simulink model "sm_worm_jack"  (R2021b)
settings: Solver=ode15s  StartTime=0.0  StopTime=15  MaxStep=0.01  RelTol=1e-3  EnableMultiTasking=on
model workspace: external: MATLAB File sm_worm_jack_parameters.m (data not in the file)
values from neighbouring files (symbols this model uses):
  ctrlStepTime = 5    [sm_worm_jack_parameters.m]
undefined symbols (not defined in the file or in its folder): jack, X, Y, Z
libraries: nesl_utility x5, sm_worm_jack_lib x4, sm_lib x3
settings Model: Creator=The MathWorks, Inc.  LastModifiedBy=The MathWorks, Inc.
settings SolverCC: AlgebraicLoopSolver=TrustRegion
settings DataIOCC: LimitDataPoints=on  ReturnWorkspaceOutputs=off
settings OptimizationCC: LifeSpan=inf
settings DebuggingCC: AllowSymbolicDim=off  SFUnexpectedBacktrackingDiag=warning  SFNoUnconditionalDefaultTransitionDiag=warning  SFExecutionAtInitializationDiag=none  SFMachineParentedDataDiag=warning  ArithmeticOperatorsInVariantConditions=warning
settings SFSimCC: SimUseLocalCustomCode=off  CustomCodeUndefinedFunction=UseInterfaceOnly
settings RTWCC: RTWUseLocalCustomCode=off
settings CodeAppCC: StateflowObjectComments=on
settings GRTTargetCC: TargetLangStandard=C89/C90 (ANSI)
settings ConfigComp: CovMetricSettings=dw  CovSaveCumulativeToWorkspaceVar=on  CovSaveSingleToWorkspaceVar=on  CovExternalEMLEnable=off  CovSFcnEnable=off
settings SimscapeCC: SimscapeNormalizeSystem=off  SimscapeLogType=all  SimscapeLogSimulationStatistics=on  SimscapeLogName=simlog_sm_worm_jack  SimscapeLogDataHistory=10000
settings ConfigurationSet: Description=SimMechanics 2G
settings ExplorerConfigSet: InternalSimMechanicsExplorerSettings="<ExplorerConfiguration><canonicalview>default</canonicalview><AnimationSetting><BasePlaybackSpeed>1.0</BasePlaybackSpeed><PlaybackSpeedFactor>1.0</PlaybackSpeedFactor></AnimationSetting><TilePanel><TileInfo><Tiles Columns=\"1\" Count=\"1\" Rows=\"1\"><Column Weight=\"1\"/><Row Weight=\"1\"/><Tile Height=\"1\" Width=\"1\" X=\"0\" Y=\"0\"/></Tiles></TileInfo><SceneInfo><SceneViewer><BGColor><R>0.60000002384185791</R><G>0.60000002384185791</G><B>0.60000002384185791</B></BGColor><Camera><DoPerspective>off</DoPerspective><Position><X>0.643732116535259746</X><Y>-0.308018560744014402</Y><Z>0.64842413062973181</Z></Position><Center><X>0.0663818473456340569</X><Y>0.269331708445611495</Y><Z>0.0710738614401060786</Z></Center><Up><X>-0.408248290463863073</X><Y>0.408248290463863073</Y><Z>0.816496580927726145</Z></Up><ViewLimDist>1</ViewLimDist><YLim>0.376296170188444967</YLim><XLim>0.50655253679213752</XLim></Camera></SceneViewer></SceneInfo></TilePanel><MechEditorPanel><Cameras/><GfxPanelCameraMap/><VideoCreator><PlaybackSpeedRatio>1.0</PlaybackSpeedRatio><FrameRate>30</FrameRate><VideoFormat>Motion JPEG AVI</VideoFormat><FrameSize>auto</FrameSize></VideoCreator></MechEditorPanel></ExplorerConfiguration>"

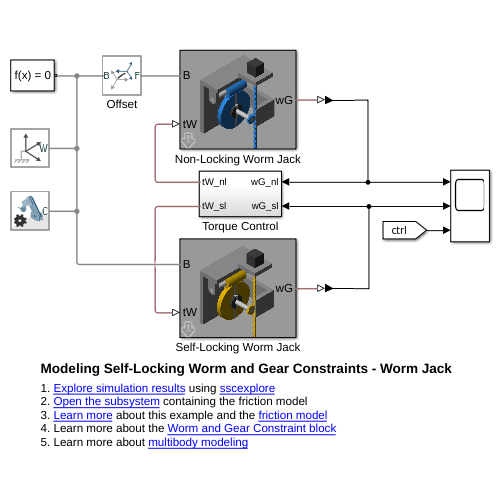
[thumbnail: Simulink's stored preview of the top-level diagram]
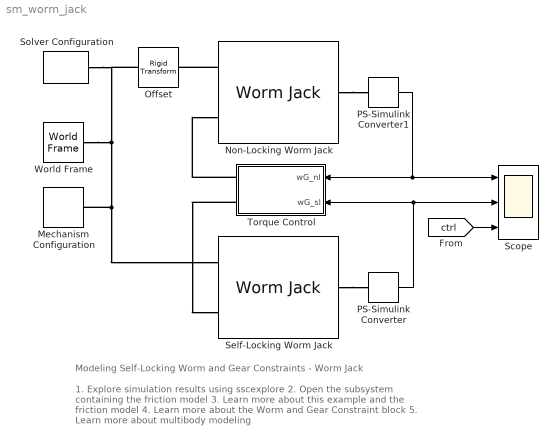
== system sm_worm_jack ==
  note: 1. Explore simulation results using sscexplore
      | 2. Open the subsystem containing the friction model
      | 3. Learn more about this example and the friction model
      | 4. Learn more about the Worm and Gear Constraint block
      | 5. Learn more about multibody modeling
  note: Modeling Self-Locking Worm and Gear Constraints - Worm Jack
  Mechanism Configuration : sm_lib/Utilities/Mechanism Configuration  UniformGravity=Constant  GravityVector=[0 0 -9.80665]  GravityUnits=m/s^2  LinearizationDelta=0.001  JointModeTransitionNonlinearIterations=2
  Non-Locking Worm Jack : sm_worm_jack_lib/Worm Jack  wormLeadAngle=nonlock.wormLeadAngle  wormRadius=jack.wormRadius  wormLength=jack.wormLength  wormShaftLength=jack.wormShaftLength  gearRadius=jack.gearRadius  gearLength=jack.gearLength  gearShaftLength=jack.gearShaftLength  collarRadius=jack.collarRadius  shaftRadius=jack.shaftRadii  rackLength=jack.rackLength  pinionRadius=jack.pinionRadius  pinionTeeth=jack.pinionTeeth  pinionShaftLength=jack.pinionShaft  loadWidth=jack.loadWidth  plateThickness=jack.plateThickness  wG_0=jack.gearRevolute_w0  muK=jack.kineticFriction  muS=jack.staticFriction  vth=jack.velocityThreshold  t_c=jack.filterConstant  wormRho=jack.wormDensity  gearRho=jack.gearDensity  shaftRho=jack.shaftDensity  collarRho=jack.collarDensity  rackRho=jack.rackDensity  pinionRho=jack.pinionDensity  housingRho=jack.housingDensity  boxRho=jack.boxDensity  wormColor=nonlock.wormColor  gearColor=nonlock.gearColor  shaftColor=jack.shaftColor  collarColor=jack.collarColor  rackColor=nonlock.rackColor  pinionColor=nonlock.pinionColor  housingColor=jack.housingColor  boxColor=jack.boxColor  sliceColor=jack.sliceColor  mask(Worm Drive Assembly){}
      settings: SourceProductBaseCode=MS
      mask Display:
      | image(imread(fullfile(matlabroot,'toolbox','physmod','sm','smdemos','worm_jack','images','sm_worm_jack_nonlocking_wormjack.png')));
      | port_label('lconn',1,'B');
      | port_label('lconn',2,'tW');
      | port_label('rconn',1,'wG');
  Offset : sm_lib/Frames and Transforms/Rigid Transform  TranslationMethod=StandardAxis  TranslationStandardOffset=nonlock.offset  TranslationLengthUnit=m  TranslationStandardAxis=+Y  TranslationCartesianOffset=0  TranslationROffset=0  TranslationROffsetUnits=m  TranslationZOffset=0  TranslationZOffsetUnits=m  TranslationThetaOffset=0  TranslationThetaOffsetUnits=deg  RotationMethod=None  RotationAngleUnits=deg  RotationStandardAxis=+Z  RotationAngle=0.0  RotationArbitraryAxis=[0 0 1]  FollAlignAxisA=+X  BaseAlignAxisA=+Y  FollAlignAxisB=+Y  BaseAlignAxisB=+Z  RotationSequenceAxes=FollowerAxes  RotationSequence=XYX  RotationSequenceAngles=[0 0 0]  RotationSequenceAnglesUnits=deg  RotationMatrix=[1 0 0; 0 1 0; 0 0 1]
  PS-Simulink Converter : nesl_utility/PS-Simulink Converter  PhysicalDomain=network_engine_domain  SubClassName=ps_output  LeftPortType=input  RightPortType=output  PseudoPeriodic=off  Frequencies=[]  Unit=deg/s  AffineConversion=off
      settings: SourceProductBaseCode=PW,SS
  PS-Simulink Converter1 : nesl_utility/PS-Simulink Converter  PhysicalDomain=network_engine_domain  SubClassName=ps_output  LeftPortType=input  RightPortType=output  PseudoPeriodic=off  Frequencies=[]  Unit=deg/s  AffineConversion=off
      settings: SourceProductBaseCode=PW,SS
  Scope : Scope  NumInputPorts=3
  Self-Locking Worm Jack : sm_worm_jack_lib/Worm Jack  wormLeadAngle=selflock.wormLeadAngle  wormRadius=jack.wormRadius  wormLength=jack.wormLength  wormShaftLength=jack.wormShaftLength  gearRadius=jack.gearRadius  gearLength=jack.gearLength  gearShaftLength=jack.gearShaftLength  collarRadius=jack.collarRadius  shaftRadius=jack.shaftRadii  rackLength=jack.rackLength  pinionRadius=jack.pinionRadius  pinionTeeth=jack.pinionTeeth  pinionShaftLength=jack.pinionShaft  loadWidth=jack.loadWidth  plateThickness=jack.plateThickness  wG_0=jack.gearRevolute_w0  muK=jack.kineticFriction  muS=jack.staticFriction  vth=jack.velocityThreshold  t_c=jack.filterConstant  wormRho=jack.wormDensity  gearRho=jack.gearDensity  shaftRho=jack.shaftDensity  collarRho=jack.collarDensity  rackRho=jack.rackDensity  pinionRho=jack.pinionDensity  housingRho=jack.housingDensity  boxRho=jack.boxDensity  wormColor=selflock.wormColor  gearColor=selflock.gearColor  shaftColor=jack.shaftColor  collarColor=jack.collarColor  rackColor=selflock.rackColor  pinionColor=selflock.pinionColor  housingColor=jack.housingColor  boxColor=jack.boxColor  sliceColor=jack.sliceColor  mask(Worm Drive Assembly){}
      settings: SourceProductBaseCode=MS
      mask Display:
      | image(imread(fullfile(matlabroot,'toolbox','physmod','sm','smdemos','worm_jack','images','sm_worm_jack_selflocking_wormjack.png')));
      | port_label('lconn',1,'B');
      | port_label('lconn',2,'tW');
      | port_label('rconn',1,'wG');
  Solver Configuration : nesl_utility/Solver Configuration  PhysicalDomain=network_engine_domain  SubClassName=solver  LeftPortType=input  RightPortType=generic  Tones=[]  Harmonics=[]  SimulateNoise=off  Profile=off  UseLocalSampling=off  EnableSwitchedLinearOptims=on  FrequencyDomain=off  UseCCode=off  RelTol=0.001  AbsTol=1e-06  MinStep=1e-09  ToWorkspace=off  RevertToSquareIcSolve=off  NumHomotopyIterations=100  PhasorMode=off  PhasorModeNumHarmonics=1  DoDC=off  ResidualTolerance=1e-9  UseLocalSolver=off  LocalSolverChoice=NE_BACKWARD_EULER_ADVANCER  LocalSolverSampleTime=0.001  DoFixedCost=off  MaxNonlinIter=3  MaxModeIter=2  ComputeImpulses=off  ImpulseIterations=2  LinearAlgebra=Sparse  EquationFormulation=NE_TIME_EF  DelaysMemoryBudget=1024  AutomaticFiltering=on  FilteringTimeConstant=0.001  PartitionStorageMethod=AS_NEEDED  PartitionMemoryBudget=1024  PartitionMethod=FAST
      settings: SourceProductBaseCode=PW,SS
  Torque Control : Subsystem
  World Frame : sm_lib/Frames and Transforms/World Frame
  wires:
  PS-Simulink Converter1/1 -> Scope/1, Torque Control/1(wG_nl)
  PS-Simulink Converter/1 -> Scope/2, Torque Control/2(wG_sl)
  [ctrl] -> Scope/3
  connections:
  Non-Locking Worm Jack/LConn1 -- Offset/RConn1
  World Frame/RConn1 -- Self-Locking Worm Jack/LConn1 -- Mechanism Configuration/RConn1 -- Offset/LConn1 -- Solver Configuration/RConn1
  Torque Control/RConn1 -- Non-Locking Worm Jack/LConn2
  Non-Locking Worm Jack/RConn1 -- PS-Simulink Converter1/LConn1
  Self-Locking Worm Jack/RConn1 -- PS-Simulink Converter/LConn1
  Torque Control/RConn2 -- Self-Locking Worm Jack/LConn2

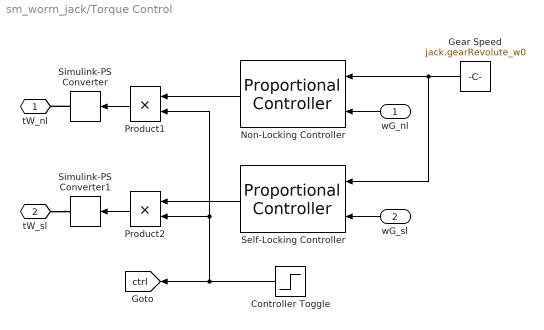
== system sm_worm_jack/Torque Control ==
  wG_nl : Inport
  wG_sl : Inport  Port=2
  Controller Toggle : Step  Time=ctrlStepTime  Before=1  After=0  SampleTime=0
  Gear Speed : Constant  Value=jack.gearRevolute_w0
  Non-Locking Controller : sm_worm_jack_lib/Proportional Controller  Kp=jack.Kp
      settings: SourceProductBaseCode=MS
  Product1 : Product
  Product2 : Product
  Self-Locking Controller : sm_worm_jack_lib/Proportional Controller  Kp=jack.Kp
      settings: SourceProductBaseCode=MS
  Simulink-PS Converter : nesl_utility/Simulink-PS Converter  PhysicalDomain=network_engine_domain  SubClassName=ps_input  LeftPortType=input  RightPortType=output  PseudoPeriodic=off  Frequencies=[]  NoiseDistribution=none  NoiseParameters=[]  Unit=1  AffineConversion=off  FilteringAndDerivatives=provide  SimscapeFilterOrder=1  InputFilterTimeConstant=0.001  UdotUserProvided=0
      settings: SourceProductBaseCode=PW,SS
  Simulink-PS Converter1 : nesl_utility/Simulink-PS Converter  PhysicalDomain=network_engine_domain  SubClassName=ps_input  LeftPortType=input  RightPortType=output  PseudoPeriodic=off  Frequencies=[]  NoiseDistribution=none  NoiseParameters=[]  Unit=1  AffineConversion=off  FilteringAndDerivatives=provide  SimscapeFilterOrder=1  InputFilterTimeConstant=0.001  UdotUserProvided=0
      settings: SourceProductBaseCode=PW,SS
  tW_nl : PMIOPort  Side=Right
  tW_sl : PMIOPort  Port=2  Side=Right
  tag scope: ctrl=global
  wires:
  Controller Toggle/1 -> Product1/2, Product2/2, [ctrl]
  wG_nl/1 -> Non-Locking Controller/2
  Gear Speed/1 -> Non-Locking Controller/1, Self-Locking Controller/1
  wG_sl/1 -> Self-Locking Controller/2
  Product1/1 -> Simulink-PS Converter/1
  Non-Locking Controller/1 -> Product1/1
  Product2/1 -> Simulink-PS Converter1/1
  Self-Locking Controller/1 -> Product2/1
  connections:
  Simulink-PS Converter/RConn1 -- tW_nl/RConn1
  tW_sl/RConn1 -- Simulink-PS Converter1/RConn1
